simulink model "vg2ex"  (Simulink 8.5)
settings: Solver=ode15s  SolverMode=SingleTasking  StartTime=0.0  StopTime=0.1  RelTol=1e-3  AbsTol=1e-6
undefined symbols (not defined in the file or in its folder): D1, Delta
libraries: powerlib x18
settings Model: Creator=PC  LastModifiedBy=PC
settings SolverCC: ZeroCrossAlgorithm=Adaptive
settings DataIOCC: LimitDataPoints=off
settings OptimizationCC: BlockReduction=off  BooleanDataType=off  ExpressionDepthLimit=128
settings DebuggingCC: SaveWithParameterizedLinksMsg=none  SignalResolutionControl=TryResolveAllWithWarning  MultiTaskDSMMsg=warning  MultiTaskCondExecSysMsg=none  FcnCallInpInsideContextMsg=EnableAllAsError  StateNameClashWarn=none
settings HardwareCC: TargetUnknown=on
settings RTWCC: TemplateMakefile=grt_vc.tmf

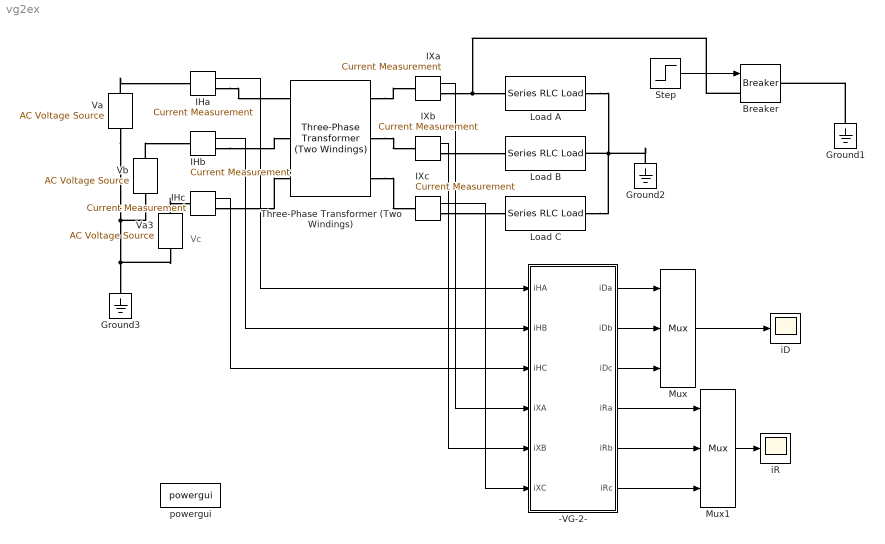
== system vg2ex ==
  note: Vc
  -VG-2- : Subsystem  mask(Transformer Masked Block){trtype=wye - delta, vector=1, Vh=13800, Vx=315000, nCTH=2400, nCTX=100}
      mask prompts: trtype "Type of Transformer"; vector "Vector Group"; Vh "Primary Voltage"; Vx "Secondry Voltage"; nCTH "CT Ratio of H"; nCTX "CT Ratio of X"
      mask help: Selection of type of transformer and vector group.
      mask init:
      | vg_20;
      mask Help: The block generates iD and iR for given input data IH, IX, each CT ratio.
      mask TypeOptions trtype: wye - delta | delta - wye | wye - wye | delta - delta
      mask TypeOptions vector: 0 | 1 | 3 | 5 | 6 | 7 | 9 | 11
      mask Display: disp(icon)
  Breaker : powerlib/Elements/Breaker  Tag=PoWeRsYsTeMbLoCk  InitialState=0  SwitchingTimes="[1/60  5/60]"  External=on  BreakerResistance=0.01  SnubberResistance=1e6  SnubberCapacitance=inf  Measurements=None  MoreParameters=on  NoBreakLoop=off
  Ground1 : powerlib/Elements/Ground  LConnTagsString=a
  Ground2 : powerlib/Elements/Ground  LConnTagsString=a
  Ground3 : powerlib/Elements/Ground  LConnTagsString=a
  IHa : powerlib/Measurements/Current Measurement  Tag=PoWeRsYsTeMmEaSuReMeNtFiRsT  PhasorSimulation=off  OutputType=Complex  PSBequivalent=0
  IHb : powerlib/Measurements/Current Measurement  Tag=PoWeRsYsTeMmEaSuReMeNt  PhasorSimulation=off  OutputType=Complex  PSBequivalent=0
  IHc : powerlib/Measurements/Current Measurement  Tag=PoWeRsYsTeMmEaSuReMeNt  PhasorSimulation=off  OutputType=Complex  PSBequivalent=0
  IXa : powerlib/Measurements/Current Measurement  Tag=PoWeRsYsTeMmEaSuReMeNt  PhasorSimulation=off  OutputType=Complex  PSBequivalent=0
  IXb : powerlib/Measurements/Current Measurement  Tag=PoWeRsYsTeMmEaSuReMeNt  PhasorSimulation=off  OutputType=Complex  PSBequivalent=0
  IXc : powerlib/Measurements/Current Measurement  Tag=PoWeRsYsTeMmEaSuReMeNt  PhasorSimulation=off  OutputType=Complex  PSBequivalent=0
  Load A : powerlib/Elements/Series RLC Load  LConnTagsString=a  RConnTagsString=__new0  NominalVoltage=1000  NominalFrequency=60  ActivePower=10e3  InductivePower=100  CapacitivePower=100  Setx0=off  InitialVoltage=0  SetiL0=off  InitialCurrent=0  Measurements=None
  Load B : powerlib/Elements/Series RLC Load  LConnTagsString=a  RConnTagsString=__new0  NominalVoltage=1000  NominalFrequency=60  ActivePower=10e3  InductivePower=100  CapacitivePower=100  Setx0=off  InitialVoltage=0  SetiL0=off  InitialCurrent=0  Measurements=None
  Load C : powerlib/Elements/Series RLC Load  LConnTagsString=a  RConnTagsString=__new0  NominalVoltage=1000  NominalFrequency=60  ActivePower=10e3  InductivePower=100  CapacitivePower=100  Setx0=off  InitialVoltage=0  SetiL0=off  InitialCurrent=0  Measurements=None
  Mux : Mux  Inputs=3
  Mux1 : Mux  Inputs=3
  Step : Step  Time=0.03
  Three-Phase Transformer (Two Windings) : powerlib/Elements/Three-Phase Transformer (Two Windings)  Winding1Connection=Yg  Winding2Connection=Delta (D1)  CoreType=Three single-phase transformers  SetSaturation=off  Hysteresis=off  DataFile='hysteresis'  SetInitialFlux=off  Measurements=None  UNITS=pu  NominalPower=[ 250e6 , 60 ]  Winding1=[ 735e3 , 0.002 , 0.08 ]  Winding2=[ 315e3 , 0.002 , 0.08 ]  Rm=500  Lm=500  L0=0.5  Saturation=[ 0,0 ; 0.0024,1.2 ; 1.0,1.52 ]  InitialFluxes=[ 0.8 , -0.8 , 0.7 ]  MoreParameters=off  BreakLoop=off  DataType=off  TransfoNumber=1
  Va : powerlib/Electrical Sources/AC Voltage Source  Tag=PoWeRsYsTeMbLoCk  Amplitude=100  Phase=0  Frequency=60  SampleTime=0  Measurements=None
  Va3 : powerlib/Electrical Sources/AC Voltage Source  Tag=PoWeRsYsTeMbLoCk  Amplitude=100  Phase=0  Frequency=60  SampleTime=0  Measurements=None
  Vb : powerlib/Electrical Sources/AC Voltage Source  Tag=PoWeRsYsTeMbLoCk  Amplitude=100  Phase=0  Frequency=60  SampleTime=0  Measurements=None
  iD : Scope
      settings: TickLabels=on  TimeRange=0.1  YMin=-0.03  YMax=0.03
  iR : Scope
      settings: TickLabels=on  YMin=-40  YMax=40
  powergui : powerlib/powergui  SimulationMode=Continuous  SolverType=Tustin/Backward Euler (TBE)  SampleTime=0  frequency=60  SPID=off  DisableSnubberDevices=off  DisableRonSwitches=off  DisableVfSwitches=off  SwTol=0  DisplayEquations=off  Interpol=off  methode=off  Ts=0  FunctionMessages=off  echomessages=off  HookPort=off  EnableUseOfTLC=off  x0status=blocks  frequencyindice=60  Pbase=100e6  ErrMax=1e-4  Iterations=50  UnitsV=kV  UnitsW=MW  buscounter=0  RestoreLinks=warning  ResistiveCurrentMeasurement=off  Frange=[0:2:500]  Ylog=off  Xlog=on  ShowGrid=off  save=off  variable=ZData  structure=0  ZoomFFT=on  StartTime=0.0  cycles=1  DisplayStyle=1  fundamental=60  FreqAxis=off  MaxFrequency=1000  frequencyindicesteady=1  RmsSteady=1  display=off
  wires:
  IHa/1 -> -VG-2-/1(iHA)
  IXc/1 -> -VG-2-/6(iXC)
  IHb/1 -> -VG-2-/2(iHB)
  IXa/1 -> -VG-2-/4(iXA)
  IHc/1 -> -VG-2-/3(iHC)
  -VG-2-/1(iDa) -> Mux/1
  -VG-2-/2(iDb) -> Mux/2
  -VG-2-/3(iDc) -> Mux/3
  Mux/1 -> iD/1
  Mux1/1 -> iR/1
  -VG-2-/4(iRa) -> Mux1/1
  -VG-2-/5(iRb) -> Mux1/2
  -VG-2-/6(iRc) -> Mux1/3
  Step/1 -> Breaker/1
  IXb/1 -> -VG-2-/5(iXB)
  connections:
  Three-Phase Transformer (Two Windings)/RConn1 -- IXa/LConn1
  Three-Phase Transformer (Two Windings)/RConn2 -- IXb/LConn1
  Three-Phase Transformer (Two Windings)/RConn3 -- IXc/LConn1
  Ground2/LConn1 -- Load A/RConn1 -- Load C/RConn1 -- Load B/RConn1
  Vb/RConn1 -- IHb/LConn1
  Va/RConn1 -- IHa/LConn1
  Va/LConn1 -- Vb/LConn1 -- Va3/LConn1 -- Ground3/LConn1
  Va3/RConn1 -- IHc/LConn1
  IHa/RConn1 -- Three-Phase Transformer (Two Windings)/LConn1
  IHb/RConn1 -- Three-Phase Transformer (Two Windings)/LConn2
  IHc/RConn1 -- Three-Phase Transformer (Two Windings)/LConn3
  IXa/RConn1 -- Breaker/LConn1 -- Load A/LConn1
  IXb/RConn1 -- Load B/LConn1
  IXc/RConn1 -- Load C/LConn1
  Ground1/LConn1 -- Breaker/RConn1

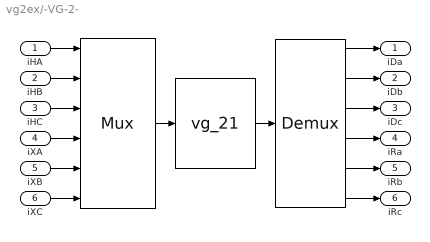
== system vg2ex/-VG-2- ==
  iHA : Inport
  iHB : Inport  Port=2
  iHC : Inport  Port=3
  iXA : Inport  Port=4
  iXB : Inport  Port=5
  iXC : Inport  Port=6
  " " : Mux  Inputs=6
  "  " : Demux  Outputs=6
  "    " : S-Function  FunctionName=vg_21  Parameters=trtype,vector,Vh,Vx,nCTH,nCTX
  iDa : Outport  InitialOutput=0
  iDb : Outport  Port=2  InitialOutput=0
  iDc : Outport  Port=3  InitialOutput=0
  iRa : Outport  Port=4  InitialOutput=0
  iRb : Outport  Port=5  InitialOutput=0
  iRc : Outport  Port=6  InitialOutput=0
  wires:
  iXC/1 -> " "/6
  "  "/6 -> iRc/1
  iXB/1 -> " "/5
  "  "/5 -> iRb/1
  iXA/1 -> " "/4
  "  "/4 -> iRa/1
  iHC/1 -> " "/3
  "  "/3 -> iDc/1
  iHB/1 -> " "/2
  "  "/2 -> iDb/1
  iHA/1 -> " "/1
  "  "/1 -> iDa/1
  "    "/1 -> "  "/1
  " "/1 -> "    "/1
